simulink model "lab1_simulink_model_2019b"  (R2019b)
settings: Solver=VariableStepAuto  StartTime=0.0  StopTime=10.0  RelTol=1e-3
undefined symbols (not defined in the file): B, fafinal, K, M
settings Model: Creator=qinqi  LastModifiedBy=qinqi
settings DataIOCC: ReturnWorkspaceOutputs=off
settings DebuggingCC: SFMachineParentedDataDiag=error

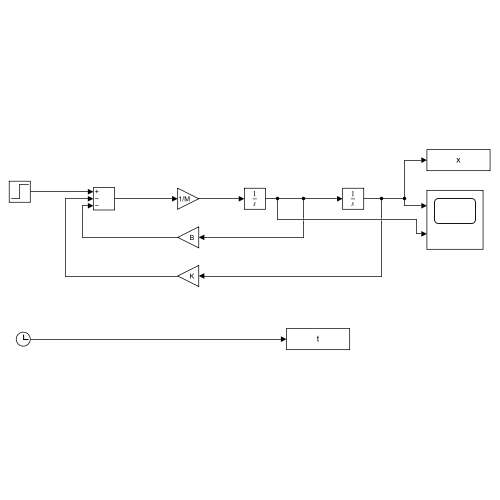
[thumbnail: Simulink's stored preview of the top-level diagram]
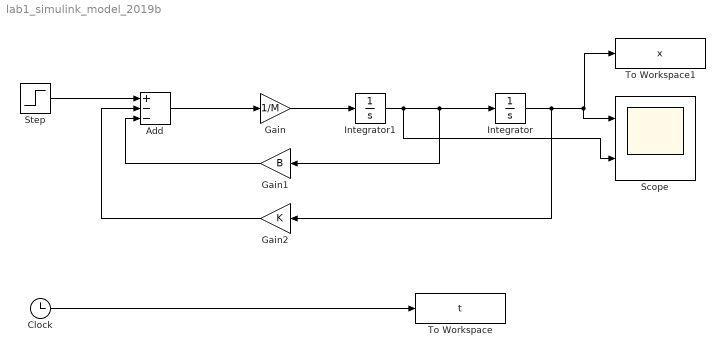
== system lab1_simulink_model_2019b ==
  Add : Sum  Inputs=+--
  Clock : Clock
  Gain : Gain  Gain=1/M
  Gain1 : Gain  Gain=B
  Gain2 : Gain  Gain=K
  Integrator : Integrator
  Integrator1 : Integrator
  Scope : Scope  NumInputPorts=2
  Step : Step  After=fafinal  SampleTime=0
  To Workspace : ToWorkspace  VariableName=t  SampleTime=-1
      settings: Save2DSignal=2-D array (concatenate along first dimension)
  To Workspace1 : ToWorkspace  VariableName=x  SampleTime=-1
      settings: Save2DSignal=2-D array (concatenate along first dimension)
  wires:
  Step/1 -> Add/1
  Add/1 -> Gain/1
  Gain/1 -> Integrator1/1
  Integrator1/1 -> Scope/2, Gain1/1, Integrator/1
  Integrator/1 -> Gain2/1, Scope/1, To Workspace1/1
  Gain1/1 -> Add/3
  Gain2/1 -> Add/2
  Clock/1 -> To Workspace/1
